simulink model "corticalBaseLine"  (Simulink 9.3)
settings: Solver=ode4  StartTime=0.0  StopTime=60  FixedStep=.004  RelTol=1e-3  EnableMultiTasking=on
Description:
  | THE MODEL IS DESIGNED BY BASABDATTA SEN BHATTACHARYA
  | AND IS AN INTELLECTUAL PROPERTY OF THE UNIVERSITY OF ULSTER,
  | NORTHERN IRELAND, UK.
  | PLEASE CITE THE FOLLOWING PAPER WHEN USING THE MODEL IN YOUR WORK:
  | Sen Bhattacharya, Basabdatta, Coyle, Damien, Maguire, Liam:
  | "A thalamo-cortico-thalamic neural mass model to study alpha rhythms in Alzheimer's
  | disease", Neural Networks (2011), doi:10.1016/j.neunet.2011.02.009.
settings Model: Creator=basabb  LastModifiedBy=alinajmaldin  SimulationMode=accelerator
settings DataIOCC: SaveOutput=off  SignalLogging=off  SaveTime=off
settings OptimizationCC: ExpressionDepthLimit=2147483647
settings DebuggingCC: SaveWithParameterizedLinksMsg=none  SolverPrmCheckMsg=warning  InheritedTsInSrcMsg=none  ModelReferenceDataLoggingMessage=none  StateNameClashWarn=warning
settings SFSimCC: SimParseCustomCode=off

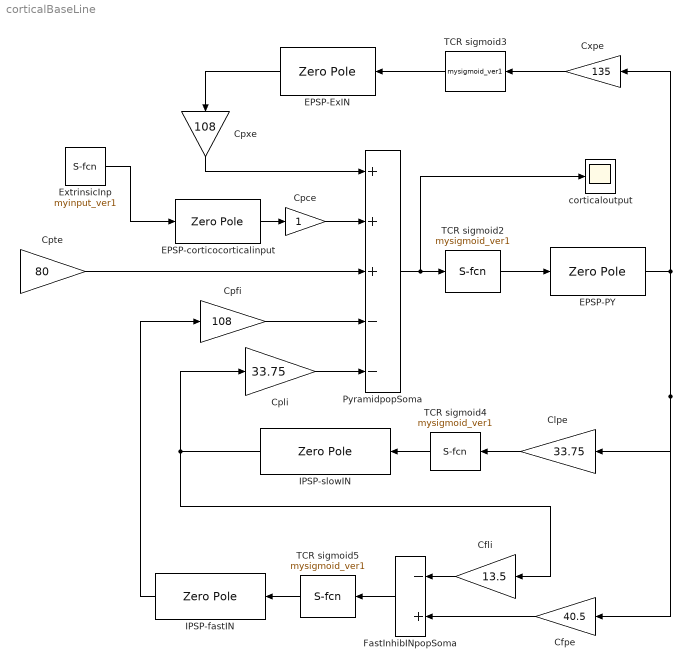
== system corticalBaseLine ==
  Cfli : Gain  Gain=13.5
  Cfpe : Gain  Gain=40.5
  Clpe : Gain  Gain=33.75
  Cpce : Gain
  Cpfi : Gain  Gain=108
  Cpli : Gain  Gain=33.75
  Cpte : Gain  Gain=80
  Cpxe : Gain  Gain=108
  Cxpe : Gain  Gain=135
  EPSP-ExIN : ZeroPole  Zeros=[]  Poles=[-40 -40]  Gain=[40* 0.0027]
  EPSP-PY : ZeroPole  Zeros=[]  Poles=[-40 -40]  Gain=[40* 0.0027]
  EPSP-corticocorticalinput : ZeroPole  Zeros=[]  Poles=[-40 -40]  Gain=[40* 0.0027]
  ExtrinsicInp : M-S-Function  Description=|  FunctionName=myinput_ver1  Parameters=30,5,60000,1
      | Input to the model with or without noise. The order of input parameters in the Dialog box is:                      
      | mean, standard deviation, length of signal,flag,constant.                                                          
      | If flag is 0, the input is a constant devoid of any noise. However, if flag is 1, the noise is added to the signal.
      mask Display: plot(312+randn(1,25))
  FastInhibINpopSoma : Sum  Inputs=-+  CollapseMode=Specified dimension  CollapseDim=4
  IPSP-fastIN : ZeroPole  Zeros=[]  Poles=[-300 -300]  Gain=[300*0.039]
  IPSP-slowIN : ZeroPole  Zeros=[]  Poles=[-20 -20]  Gain=[20*0.0045]
  PyramidpopSoma : Sum  Inputs=+++--  CollapseMode=Specified dimension  CollapseDim=4
  TCR sigmoid{2..5} (4 alike) : M-S-Function  FunctionName=mysigmoid_ver1  Parameters=2.5,560,0.006
      mask Display: plot(1./(1+exp(-0.75.*([1:25]-12))))
  corticaloutput : Scope
  wires:
  PyramidpopSoma/1 -> TCR sigmoid2/1, corticaloutput/1
  TCR sigmoid2/1 -> EPSP-PY/1
  Cxpe/1 -> TCR sigmoid3/1
  TCR sigmoid3/1 -> EPSP-ExIN/1
  Clpe/1 -> TCR sigmoid4/1
  TCR sigmoid4/1 -> IPSP-slowIN/1
  IPSP-slowIN/1 -> Cpli/1, Cfli/1
  Cfli/1 -> FastInhibINpopSoma/1
  TCR sigmoid5/1 -> IPSP-fastIN/1
  IPSP-fastIN/1 -> Cpfi/1
  EPSP-ExIN/1 -> Cpxe/1
  EPSP-PY/1 -> Clpe/1, Cfpe/1, Cxpe/1
  FastInhibINpopSoma/1 -> TCR sigmoid5/1
  Cfpe/1 -> FastInhibINpopSoma/2
  ExtrinsicInp/1 -> EPSP-corticocorticalinput/1
  Cpxe/1 -> PyramidpopSoma/1
  EPSP-corticocorticalinput/1 -> Cpce/1
  Cpfi/1 -> PyramidpopSoma/4
  Cpli/1 -> PyramidpopSoma/5
  Cpte/1 -> PyramidpopSoma/3
  Cpce/1 -> PyramidpopSoma/2
